simulink model "FCS_SIL"  (R2025b)
settings: Solver=ode3  StartTime=0.0  StopTime=10.0  RelTol=1e-3
PostLoadFcn:
  | Init
InitFcn:
  | Init
undefined symbols (not defined in the file): DWORK0, DWORK1, DWORK10, DWORK11, DWORK12, DWORK13, DWORK14, DWORK15, DWORK16, DWORK17, DWORK18, DWORK19, DWORK2, DWORK20, DWORK21, DWORK22, DWORK23, DWORK24, DWORK3, DWORK4, DWORK5, DWORK6, DWORK7, DWORK8, DWORK9
settings Model: Creator=1manu  LastModifiedBy=1manu
settings DataIOCC: SaveOutput=off  SaveTime=off
settings OptimizationCC: DefaultParameterBehavior=Inlined

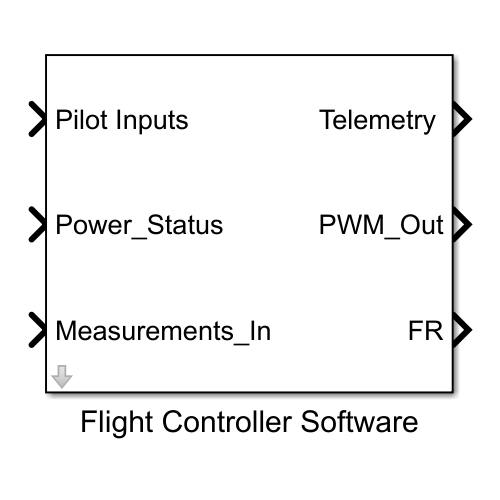
[thumbnail: Simulink's stored preview of the top-level diagram]
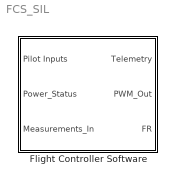
== system FCS_SIL ==
  Flight Controller Software : Subsystem
      mask help: Simulink:masks:GenSFuncDesc_MD
      mask Help: eval('feval(''rtwprivate'',''rtwhelpview'',''rtw_sfcn_block'')');

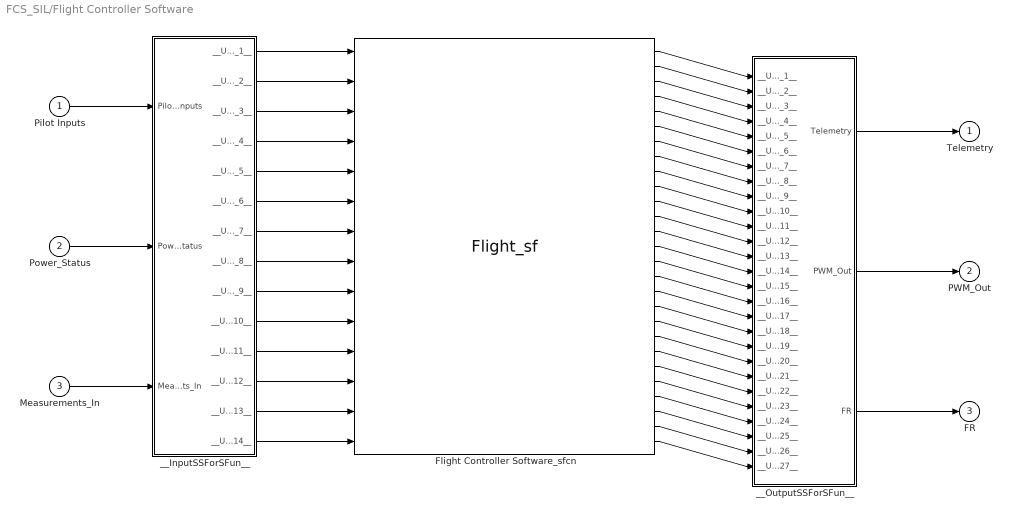
== system FCS_SIL/Flight Controller Software ==
  Pilot Inputs : Inport
  Power_Status : Inport  Port=2
  Measurements_In : Inport  Port=3
  Flight Controller Software_sfcn : S-Function  FunctionName=Flight_sf  SFunctionModules=""  SFunctionDeploymentMode=off  EnableBusSupport=off  SFcnStateName=DWORK0,DWORK1,DWORK2,DWORK3,DWORK4,DWORK5,DWORK6,DWORK7,DWORK8,DWORK9,DWORK10,DWORK11,DWORK12,DWORK13,DWORK14,DWORK15,DWORK16,DWORK17,DWORK18,DWORK19,DWORK20,DWORK21,DWORK22,DWORK23,DWORK24  mask{rtw_sf_name=Flight_sf, showVar=off}
      mask prompts: rtw_sf_name "Simulink:masks:GenSFuncName_MP"; showVar "Simulink:masks:GenSFuncShowModuleList_MP"
      mask help: Simulink:masks:GenSFuncDesc_MD
      mask init:
      | displist = '';
      | if ~strcmp(get_param(gcb, 'FunctionName'), rtw_sf_name);
      |   set_param(gcb, 'FunctionName', rtw_sf_name);
      | end
      | % Check if we are generating code
      | rtw_mode = false;
      | if strcmpi(get_param(bdroot(gcb),'SimulationStatus'),'Initializing')
      | 	rtw_mode = strcmpi(get_param(bdroot(gcb),'BuildingRTWCode'),'on') && ...
      | 		~strcmpi(get_param(bdroot(gcb),'TargetStyle'),'SimulationTarget');
      | end
      | if showVar || rtw_mode
      | 	if exist('rtwsfunc') == 2 | exist('rtwsfunc') == 6
      | 		tmplist = rtwsfunc(rtw_sf_name,gcb);
      | 		tmplist = DAStudio.message('Simulink:masks:GenSFuncListOfModules_IC', tmplist);
      | 	elseif showVar
      | 		tmplist1 = DAStudio.message('Simulink:masks:GenSFuncListOfModules_IC', '');
      |         tmplist2 = DAStudio.message('Simulink:masks:GenSFuncNotLicensed_IC');
      |         tmplist = [tmplist1 tmplist2];
      |  	end
      | end
      | if showVar
      |   displist = tmplist;
      | end
      settings: SFcnIsStateOwnerBlock=on
      settings: CopyFcn=|
      | if ~strcmp(get_param(gcb,'Linkstatus'),'none') && ...
      | ~strcmp(get_param(gcb,'Linkstatus'),'implicit')
      |   set_param(gcb,'LinkStatus','none');
      | end
      mask Help: eval('feval(''rtwprivate'',''rtwhelpview'',''rtw_sfcn_block'')');
      mask Display:
      | port_label('input',1,'Roll');
      | port_label('input',2,'Pitch');
      | port_label('input',3,'Yaw');
      | port_label('input',4,'Throttle');
      | port_label('input',5,'Arm/Disarm');
      | port_label('input',6,'Mode');
      | port_label('input',7,'Volt');
      | port_label('input',8,'Curr');
      | port_label('input',9,'Ve_m');
      | port_label('input',10,'Xe_m');
      | port_label('input',11,'z_m');
      | port_label('input',12,'Mag_m');
      | port_label('input',13,'Wb_m');
      | port_label('input',14,'Acc_m');
      | port_label('output',1,'ALT');
      | port_label('output',2,'VS');
      | port_label('output',3,'SPEED');
      | port_label('output',4,'COMPASS');
      | port_label('output',5,'STATUS');
      | port_label('output',6,'MODE');
      | port_label('output',7,'TIMER');
      | port_label('output',8,'BAT PER');
      | port_label('output',9,'BAT VOLT');
      | port_label('output',10,'PWM_1');
      | port_label('output',11,'PWM_2');
      | port_label('output',12,'PWM_3');
      | port_label('output',13,'PWM_4');
      | port_label('output',14,'PWM_1b');
      | port_label('output',15,'PWM_2b');
      | port_label('output',16,'PWM_3b');
      | port_label('output',17,'PWM_4b');
      | port_label('output',18,'PWM_1a');
      | port_label('output',19,'PWM_2a');
      | port_label('output',20,'PWM_4a');
      | port_label('output',21,'PWM_3a');
      | port_label('output',22,'Vel');
      | port_label('output',23,'Pos');
      | port_label('output',24,'Angles');
      | port_label('output',25,'Rates');
      | port_label('output',26,'System Status');
      | port_label('output',27,'Setpoints');
  __InputSSForSFun__ : Subsystem
  __OutputSSForSFun__ : Subsystem
  "Telemetry " : Outport
  PWM_Out : Outport  Port=2
  FR : Outport  Port=3
  wires:
  Pilot Inputs/1 -> __InputSSForSFun__/1(Pilot Inputs)
  Power_Status/1 -> __InputSSForSFun__/2(Power_Status)
  Measurements_In/1 -> __InputSSForSFun__/3(Measurements_In)
  __InputSSForSFun__/1(__UniqueOutportName__1__) -> Flight Controller Software_sfcn/1
  __InputSSForSFun__/2(__UniqueOutportName__2__) -> Flight Controller Software_sfcn/2
  __InputSSForSFun__/3(__UniqueOutportName__3__) -> Flight Controller Software_sfcn/3
  __InputSSForSFun__/4(__UniqueOutportName__4__) -> Flight Controller Software_sfcn/4
  __InputSSForSFun__/5(__UniqueOutportName__5__) -> Flight Controller Software_sfcn/5
  __InputSSForSFun__/6(__UniqueOutportName__6__) -> Flight Controller Software_sfcn/6
  __InputSSForSFun__/7(__UniqueOutportName__7__) -> Flight Controller Software_sfcn/7
  __InputSSForSFun__/8(__UniqueOutportName__8__) -> Flight Controller Software_sfcn/8
  __InputSSForSFun__/9(__UniqueOutportName__9__) -> Flight Controller Software_sfcn/9
  __InputSSForSFun__/10(__UniqueOutportName__10__) -> Flight Controller Software_sfcn/10
  __InputSSForSFun__/11(__UniqueOutportName__11__) -> Flight Controller Software_sfcn/11
  __InputSSForSFun__/12(__UniqueOutportName__12__) -> Flight Controller Software_sfcn/12
  __InputSSForSFun__/13(__UniqueOutportName__13__) -> Flight Controller Software_sfcn/13
  __InputSSForSFun__/14(__UniqueOutportName__14__) -> Flight Controller Software_sfcn/14
  Flight Controller Software_sfcn/1 -> __OutputSSForSFun__/1(__UniqueInportName__1__)
  Flight Controller Software_sfcn/2 -> __OutputSSForSFun__/2(__UniqueInportName__2__)
  Flight Controller Software_sfcn/3 -> __OutputSSForSFun__/3(__UniqueInportName__3__)
  Flight Controller Software_sfcn/4 -> __OutputSSForSFun__/4(__UniqueInportName__4__)
  Flight Controller Software_sfcn/5 -> __OutputSSForSFun__/5(__UniqueInportName__5__)
  Flight Controller Software_sfcn/6 -> __OutputSSForSFun__/6(__UniqueInportName__6__)
  Flight Controller Software_sfcn/7 -> __OutputSSForSFun__/7(__UniqueInportName__7__)
  Flight Controller Software_sfcn/8 -> __OutputSSForSFun__/8(__UniqueInportName__8__)
  Flight Controller Software_sfcn/9 -> __OutputSSForSFun__/9(__UniqueInportName__9__)
  Flight Controller Software_sfcn/10 -> __OutputSSForSFun__/10(__UniqueInportName__10__)
  Flight Controller Software_sfcn/11 -> __OutputSSForSFun__/11(__UniqueInportName__11__)
  Flight Controller Software_sfcn/12 -> __OutputSSForSFun__/12(__UniqueInportName__12__)
  Flight Controller Software_sfcn/13 -> __OutputSSForSFun__/13(__UniqueInportName__13__)
  Flight Controller Software_sfcn/14 -> __OutputSSForSFun__/14(__UniqueInportName__14__)
  Flight Controller Software_sfcn/15 -> __OutputSSForSFun__/15(__UniqueInportName__15__)
  Flight Controller Software_sfcn/16 -> __OutputSSForSFun__/16(__UniqueInportName__16__)
  Flight Controller Software_sfcn/17 -> __OutputSSForSFun__/17(__UniqueInportName__17__)
  Flight Controller Software_sfcn/18 -> __OutputSSForSFun__/18(__UniqueInportName__18__)
  Flight Controller Software_sfcn/19 -> __OutputSSForSFun__/19(__UniqueInportName__19__)
  Flight Controller Software_sfcn/20 -> __OutputSSForSFun__/20(__UniqueInportName__20__)
  Flight Controller Software_sfcn/21 -> __OutputSSForSFun__/21(__UniqueInportName__21__)
  Flight Controller Software_sfcn/22 -> __OutputSSForSFun__/22(__UniqueInportName__22__)
  Flight Controller Software_sfcn/23 -> __OutputSSForSFun__/23(__UniqueInportName__23__)
  Flight Controller Software_sfcn/24 -> __OutputSSForSFun__/24(__UniqueInportName__24__)
  Flight Controller Software_sfcn/25 -> __OutputSSForSFun__/25(__UniqueInportName__25__)
  Flight Controller Software_sfcn/26 -> __OutputSSForSFun__/26(__UniqueInportName__26__)
  Flight Controller Software_sfcn/27 -> __OutputSSForSFun__/27(__UniqueInportName__27__)
  __OutputSSForSFun__/1("Telemetry ") -> "Telemetry "/1
  __OutputSSForSFun__/2(PWM_Out) -> PWM_Out/1
  __OutputSSForSFun__/3(FR) -> FR/1

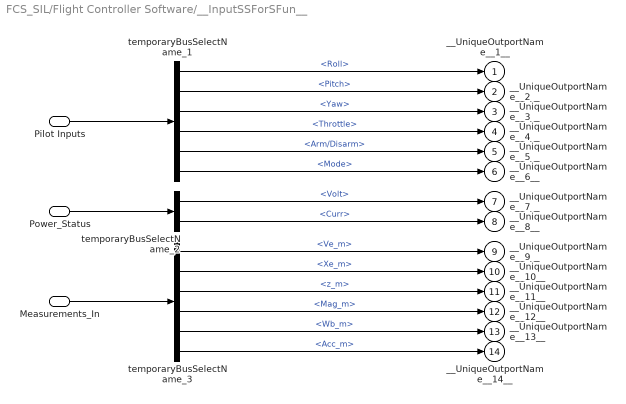
== system FCS_SIL/Flight Controller Software/__InputSSForSFun__ ==
  Pilot Inputs : Inport
  Power_Status : Inport  Port=2
  Measurements_In : Inport  Port=3
  temporaryBusSelectName_1 : BusSelector  OutputSignals=Roll,Pitch,Yaw,Throttle,Arm/Disarm,Mode
  temporaryBusSelectName_2 : BusSelector  OutputSignals=Volt,Curr
  temporaryBusSelectName_3 : BusSelector  OutputSignals=Ve_m,Xe_m,z_m,Mag_m,Wb_m,Acc_m
  __UniqueOutportName__1__ : Outport
  __UniqueOutportName__2__ : Outport  Port=2
  __UniqueOutportName__3__ : Outport  Port=3
  __UniqueOutportName__4__ : Outport  Port=4
  __UniqueOutportName__5__ : Outport  Port=5
  __UniqueOutportName__6__ : Outport  Port=6
  __UniqueOutportName__7__ : Outport  Port=7
  __UniqueOutportName__8__ : Outport  Port=8
  __UniqueOutportName__9__ : Outport  Port=9
  __UniqueOutportName__10__ : Outport  Port=10
  __UniqueOutportName__11__ : Outport  Port=11
  __UniqueOutportName__12__ : Outport  Port=12
  __UniqueOutportName__13__ : Outport  Port=13
  __UniqueOutportName__14__ : Outport  Port=14
  wires:
  Pilot Inputs/1 -> temporaryBusSelectName_1/1
  Power_Status/1 -> temporaryBusSelectName_2/1
  Measurements_In/1 -> temporaryBusSelectName_3/1
  temporaryBusSelectName_1/1 -> __UniqueOutportName__1__/1  "<Roll>"
  temporaryBusSelectName_1/2 -> __UniqueOutportName__2__/1  "<Pitch>"
  temporaryBusSelectName_1/3 -> __UniqueOutportName__3__/1  "<Yaw>"
  temporaryBusSelectName_1/4 -> __UniqueOutportName__4__/1  "<Throttle>"
  temporaryBusSelectName_1/5 -> __UniqueOutportName__5__/1  "<Arm/Disarm>"
  temporaryBusSelectName_1/6 -> __UniqueOutportName__6__/1  "<Mode>"
  temporaryBusSelectName_2/1 -> __UniqueOutportName__7__/1  "<Volt>"
  temporaryBusSelectName_2/2 -> __UniqueOutportName__8__/1  "<Curr>"
  temporaryBusSelectName_3/1 -> __UniqueOutportName__9__/1  "<Ve_m>"
  temporaryBusSelectName_3/2 -> __UniqueOutportName__10__/1  "<Xe_m>"
  temporaryBusSelectName_3/3 -> __UniqueOutportName__11__/1  "<z_m>"
  temporaryBusSelectName_3/4 -> __UniqueOutportName__12__/1  "<Mag_m>"
  temporaryBusSelectName_3/5 -> __UniqueOutportName__13__/1  "<Wb_m>"
  temporaryBusSelectName_3/6 -> __UniqueOutportName__14__/1  "<Acc_m>"

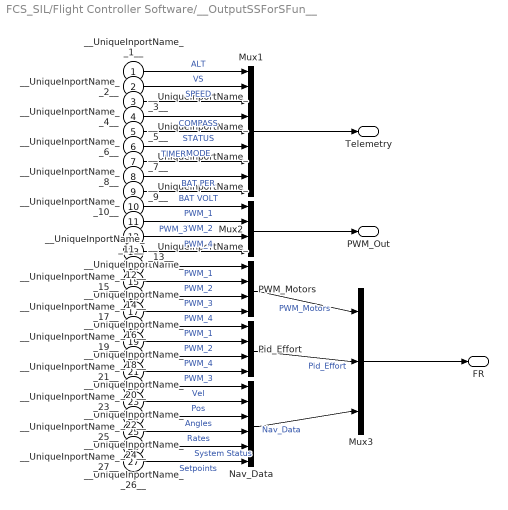
== system FCS_SIL/Flight Controller Software/__OutputSSForSFun__ ==
  __UniqueInportName__1__ : Inport
  __UniqueInportName__2__ : Inport  Port=2
  __UniqueInportName__3__ : Inport  Port=3
  __UniqueInportName__4__ : Inport  Port=4
  __UniqueInportName__5__ : Inport  Port=5
  __UniqueInportName__6__ : Inport  Port=6
  __UniqueInportName__7__ : Inport  Port=7
  __UniqueInportName__8__ : Inport  Port=8
  __UniqueInportName__9__ : Inport  Port=9
  __UniqueInportName__10__ : Inport  Port=10
  __UniqueInportName__11__ : Inport  Port=11
  __UniqueInportName__12__ : Inport  Port=12
  __UniqueInportName__13__ : Inport  Port=13
  __UniqueInportName__14__ : Inport  Port=14
  __UniqueInportName__15__ : Inport  Port=15
  __UniqueInportName__16__ : Inport  Port=16
  __UniqueInportName__17__ : Inport  Port=17
  __UniqueInportName__18__ : Inport  Port=18
  __UniqueInportName__19__ : Inport  Port=19
  __UniqueInportName__20__ : Inport  Port=20
  __UniqueInportName__21__ : Inport  Port=21
  __UniqueInportName__22__ : Inport  Port=22
  __UniqueInportName__23__ : Inport  Port=23
  __UniqueInportName__24__ : Inport  Port=24
  __UniqueInportName__25__ : Inport  Port=25
  __UniqueInportName__26__ : Inport  Port=26
  __UniqueInportName__27__ : Inport  Port=27
  Mux1 : BusCreator  Inputs=9
  Mux2 : BusCreator  Inputs=4
  Mux3 : BusCreator  Inputs=3
  Nav_Data : BusCreator  Inputs=6
  PWM_Motors : BusCreator  Inputs=4
  Pid_Effort : BusCreator  Inputs=4
  "Telemetry " : Outport
  PWM_Out : Outport  Port=2
  FR : Outport  Port=3
  wires:
  __UniqueInportName__1__/1 -> Mux1/1  "ALT"
  __UniqueInportName__2__/1 -> Mux1/2  "VS"
  __UniqueInportName__3__/1 -> Mux1/3  "SPEED"
  __UniqueInportName__4__/1 -> Mux1/4  "COMPASS"
  __UniqueInportName__5__/1 -> Mux1/5  "STATUS"
  __UniqueInportName__6__/1 -> Mux1/6  "MODE"
  __UniqueInportName__7__/1 -> Mux1/7  "TIMER"
  __UniqueInportName__8__/1 -> Mux1/8  "BAT PER"
  __UniqueInportName__9__/1 -> Mux1/9  "BAT VOLT"
  Mux1/1 -> "Telemetry "/1
  __UniqueInportName__10__/1 -> Mux2/1  "PWM_1"
  __UniqueInportName__11__/1 -> Mux2/2  "PWM_2"
  __UniqueInportName__12__/1 -> Mux2/3  "PWM_3"
  __UniqueInportName__13__/1 -> Mux2/4  "PWM_4"
  Mux2/1 -> PWM_Out/1
  __UniqueInportName__14__/1 -> PWM_Motors/1  "PWM_1"
  __UniqueInportName__15__/1 -> PWM_Motors/2  "PWM_2"
  __UniqueInportName__16__/1 -> PWM_Motors/3  "PWM_3"
  __UniqueInportName__17__/1 -> PWM_Motors/4  "PWM_4"
  __UniqueInportName__18__/1 -> Pid_Effort/1  "PWM_1"
  __UniqueInportName__19__/1 -> Pid_Effort/2  "PWM_2"
  __UniqueInportName__20__/1 -> Pid_Effort/3  "PWM_4"
  __UniqueInportName__21__/1 -> Pid_Effort/4  "PWM_3"
  __UniqueInportName__22__/1 -> Nav_Data/1  "Vel"
  __UniqueInportName__23__/1 -> Nav_Data/2  "Pos"
  __UniqueInportName__24__/1 -> Nav_Data/3  "Angles"
  __UniqueInportName__25__/1 -> Nav_Data/4  "Rates"
  __UniqueInportName__26__/1 -> Nav_Data/5  "System Status"
  __UniqueInportName__27__/1 -> Nav_Data/6  "Setpoints"
  PWM_Motors/1 -> Mux3/1  "PWM_Motors"
  Pid_Effort/1 -> Mux3/2  "Pid_Effort"
  Nav_Data/1 -> Mux3/3  "Nav_Data"
  Mux3/1 -> FR/1
